simulink subsystem "Torque_Vectoring_2WD_NO_FILTER_NO_REGEN"  (R2023b)
settings: Solver=VariableStepAuto  StartTime=0.0  StopTime=10.0  RelTol=1e-3
undefined symbols (not defined in the file): dIb, half_track, I_FUSE, k_TL, PLb, r_power_sat, s, Tmc, Tmo, v, yaw_table
libraries: simulink x1
settings Model: Creator=Inver  LastModifiedBy=Inver
settings SFSimCC: SimCustomHeaderCode="#include \"simplex.h\""  SimUserSources=Code_Generation_Project/simplex.c

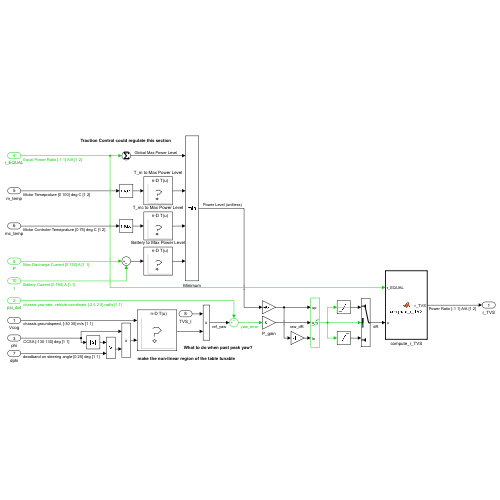
[thumbnail: Simulink's stored preview of the top-level diagram]
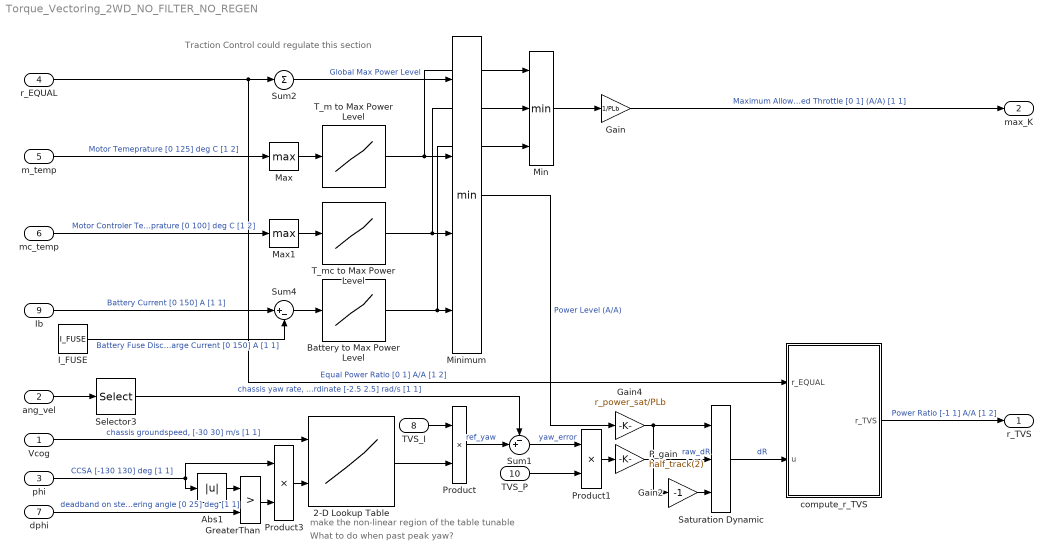
== system Torque_Vectoring_2WD_NO_FILTER_NO_REGEN ==
  note: What to do when past peak yaw?
  note: make the non-linear region of the table tunable
  note: Traction Control could regulate this section
  Vcog : Inport
  ang_vel : Inport  Port=2  OutDataTypeStr=double  LockScale=on
  phi : Inport  Port=3
  r_EQUAL : Inport  Port=4  OutDataTypeStr=double  LockScale=on
  m_temp : Inport  Port=5
  mc_temp : Inport  Port=6
  dphi : Inport  Port=7
  TVS_I : Inport  Port=8
  Ib : Inport  Port=9  OutDataTypeStr=double  LockScale=on
  TVS_P : Inport  Port=10
  2-D Lookup Table : Lookup_n-D  BreakpointsForDimension1=v  BreakpointsForDimension2=s  IndexSearchMethod=Evenly spaced points  Table=yaw_table  ExtrapMethod=Clip  RemoveProtectionInput=on  UseLastTableValue=on  InternalRulePriority=Speed  RndMeth=Simplest
      settings: InputPortMap=u0,u1
  Abs1 : Abs  SaturateOnIntegerOverflow=off
  Battery to Max Power Level : Lookup_n-D  NumberOfTableDimensions=1  LookupTableObject=''  BreakpointsForDimension1=dIb  BreakpointsForDimension1FirstPoint=10  BreakpointsForDimension2FirstPoint=10  BreakpointsForDimension1Spacing=12  BreakpointsForDimension2Spacing=12  IndexSearchMethod=Evenly spaced points  Table=k_TL  ExtrapMethod=Clip  RemoveProtectionInput=on  UseLastTableValue=on  InternalRulePriority=Speed  RndMeth=Simplest
  Gain : Gain  Gain=1/PLb
  Gain2 : Gain  Gain=-1
  Gain4 : Gain  Gain=r_power_sat/PLb
  GreaterThan : RelationalOperator  Operator=>  OutDataTypeStr=boolean  RndMeth=Simplest  InputSameDT=off
  I_FUSE : Constant  Value=I_FUSE
  Max : MinMax  Function=max
  Max1 : MinMax  Function=max
  Min : MinMax  Inputs=3
  Minimum : MinMax  Inputs=4
  P_gain : Gain  Gain=half_track(2)  ParamDataTypeStr=double  OutDataTypeStr=double
  Product : Product  OutDataTypeStr=Inherit: Inherit via back propagation
  Product1 : Product
  Product3 : Product
  Saturation Dynamic : simulink/Discontinuities/Saturation Dynamic  OutMin=[]  OutMax=[]  OutDataTypeStr=Inherit: Same as second input  OutDataType=fixdt(1, 16)  OutScaling=2^-10  DoSatur=off
  Selector3 : Selector  IndexMode=Zero-based  InputPortWidth=3  IndexOptions=Index vector (dialog)  Indices=2  OutputSizes=1
  Sum1 : Sum  Inputs=-+|  OutDataTypeStr=Inherit: Inherit via back propagation
  Sum2 : Sum  Inputs=+
  Sum4 : Sum  Inputs=|+-
  T_m to Max Power Level : Lookup_n-D  NumberOfTableDimensions=1  BreakpointsForDimension1=Tmo  IndexSearchMethod=Evenly spaced points  Table=k_TL  ExtrapMethod=Clip  RemoveProtectionInput=on  UseLastTableValue=on  InternalRulePriority=Speed  RndMeth=Simplest
  T_mc to Max Power Level : Lookup_n-D  NumberOfTableDimensions=1  BreakpointsForDimension1=Tmc  IndexSearchMethod=Evenly spaced points  Table=k_TL  ExtrapMethod=Clip  RemoveProtectionInput=on  UseLastTableValue=on  InternalRulePriority=Speed  RndMeth=Simplest
  compute_r_TVS : MATLAB Function  TreatAsAtomicUnit=on
  r_TVS : Outport
  max_K : Outport  Port=2
  wires:
  Sum4/1 -> Battery to Max Power Level/1
  Ib/1 -> Sum4/1  "Battery Current [0 150] A [1 1]"
  Battery to Max Power Level/1 -> Minimum/4, Min/3
  I_FUSE/1 -> Sum4/2  "Battery Fuse Discharge Current [0 150] A [1 1]"
  Product3/1 -> 2-D Lookup Table/2
  Sum2/1 -> Minimum/1  "Global Max Power Level"
  phi/1 -> Abs1/1, Product3/1  "CCSA [-130 130] deg [1 1]"
  Saturation Dynamic/1 -> compute_r_TVS/2(u)  "dR"
  m_temp/1 -> Max/1  "Motor Temeprature [0 125] deg C [1 2]"
  r_EQUAL/1 -> Sum2/1, compute_r_TVS/1(r_EQUAL)  "Equal Power Ratio [0 1] A/A [1 2]"
  Minimum/1 -> Gain4/1  "Power Level (A/A)"
  Vcog/1 -> 2-D Lookup Table/1  "chassis groundspeed, [-30 30] m/s [1 1]"
  mc_temp/1 -> Max1/1  "Motor Controler Temeprature [0 100] deg C [1 2]"
  Max1/1 -> T_mc to Max Power Level/1
  T_m to Max Power Level/1 -> Minimum/2, Min/1
  T_mc to Max Power Level/1 -> Minimum/3, Min/2
  Max/1 -> T_m to Max Power Level/1
  TVS_I/1 -> Product/1
  Product/1 -> Sum1/2  "ref_yaw"
  ang_vel/1 -> Selector3/1
  2-D Lookup Table/1 -> Product/2
  GreaterThan/1 -> Product3/2
  Abs1/1 -> GreaterThan/1
  Sum1/1 -> Product1/1  "yaw_error"
  Gain2/1 -> Saturation Dynamic/3
  Gain4/1 -> Saturation Dynamic/1, Gain2/1
  dphi/1 -> GreaterThan/2  "deadband on steering angle [0 25] deg [1 1]"
  P_gain/1 -> Saturation Dynamic/2  "raw_dR"
  compute_r_TVS/1(r_TVS) -> r_TVS/1  "Power Ratio [-1 1] A/A [1 2]"
  Selector3/1 -> Sum1/1  "chassis yaw rate, vehicle coordinate [-2.5 2.5] rad/s [1 1]"
  TVS_P/1 -> Product1/2
  Product1/1 -> P_gain/1
  Min/1 -> Gain/1
  Gain/1 -> max_K/1  "Maximum Allowed Throttle [0 1] (A/A) [1 1]"

== matlab function Torque_Vectoring_2WD_NO_FILTER_NO_REGEN/compute_r_TVS ==
  data: r_EQUAL input; u input; r_TVS output
function r_TVS = compute_r_TVS(r_EQUAL,u)
    if u > 0
        r_TVS = [r_EQUAL(1) r_EQUAL(1)-abs(u)];
    else
        r_TVS = [r_EQUAL(1)-abs(u) r_EQUAL(1)];
    end
end
